simulink subsystem "Communication_Simulator"  (R2024a)
settings: Solver=VariableStepAuto  StartTime=0.0  StopTime=10.0  RelTol=1e-3
undefined symbols (not defined in the file): paramRFSatLink, QAM, rfSatSourceSamplesPerSymbol, rfSatSourceSampleTime
libraries: commrflib2 x24, dspsigops x12, commrfcorlib x8, commfilt2 x8, commdigbbndam3 x8, dspsolvers x8, simulink x8, commrandsrc3 x4, commsink2 x4, commdemoslib x4, impairlib x4, commsync2 x4
(part 1 of 3)
settings Model: Creator=dani  LastModifiedBy=dani

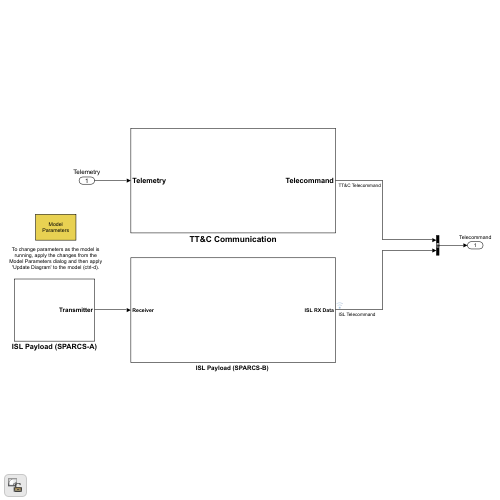
[thumbnail: Simulink's stored preview of the top-level diagram]
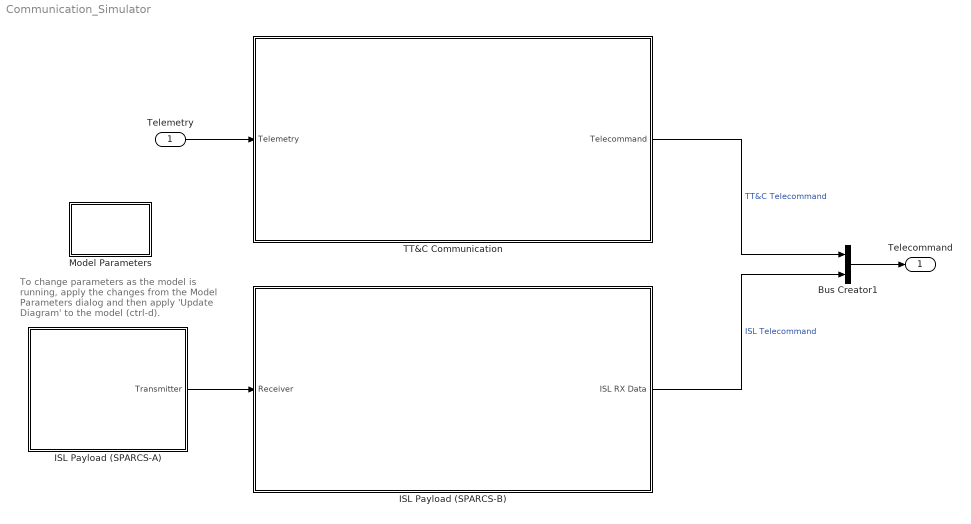
== system Communication_Simulator ==
  note: To change parameters as the model is running, apply the changes from the Model Parameters dialog and then apply 'Update Diagram' to the model (ctrl-d).
  Telemetry : Inport
  Bus Creator1 : BusCreator  Inputs=2
  ISL Payload (SPARCS-A) : Subsystem
  "ISL Payload (SPARCS-B) " : Subsystem
  Model Parameters : Subsystem  mask(Model Parameters){altitude=2500, frequency=435, antDiam=[.4 .4], selTemp=0 (no noise), selLvlBO=30 dB  (negligible nonlinearity), selDoppler=0 Hz, selNoPh=Negligible (-100 dBc/Hz @ 100 Hz), selImbal=None, selADC=No ADC, selPreDistortion=off, selDcOffset=off, selCorrIQ=off, selCorrDoppler=off}
      mask prompts: altitude "Satellite altitude (km):"; frequency "Frequency (MHz):"; antDiam "Transmit and receive antenna diameters (m):"; selTemp "Noise temperature (K):"; selLvlBO "HPA backoff level:"; selDoppler "Doppler error:"; selNoPh "Phase noise:"; selImbal "I/Q imbalance and DC offset:"; selADC "ADC:"; selPreDistortion "Digital predistortion"; selDcOffset "DC offset correction"; selCorrIQ "I/Q imbalance correction"; selCorrDoppler "Doppler correction"
      mask help:
      | Select the scenarios from the mask to change the link parameters. Each of the mask parameters sets the parameters in the corresponding RF impairment or corresponding correction block(s).
      |
      | To make changes as the model is running, apply the changes from this dialog and then apply Update Diagram to the model (crtl-d).
      mask init:
      | commrfsatlink_mask(selLvlBO,selTemp, ...
      |     selDoppler, selImbal, selNoPh, ...
      |     selDcOffset, selCorrDoppler, selCorrIQ, altitude, ...
      |     frequency, antDiam,8,6,selPreDistortion,selADC);
      mask Help: helpview(commdhelp);
      mask TypeOptions selTemp: 0 (no noise) | 20 (very low noise level) | 290 (typical noise level) | 500 (high noise level)
      mask TypeOptions selLvlBO: 30 dB  (negligible nonlinearity) | 7 dB  (moderate nonlinearity) | 1 dB  (severe nonlinearity)
      mask TypeOptions selDoppler: 0 Hz | 3 Hz
      mask TypeOptions selNoPh: Negligible (-100 dBc/Hz @ 100 Hz) | Low  (-55 dBc/Hz @ 100 Hz) | High  (-48 dBc/Hz @ 100 Hz)
      mask TypeOptions selImbal: None | Amplitude imbalance (3 dB) | Phase imbalance (20 deg) | In-phase DC offset (1e-8) | Quadrature DC offset (5e-8)
      mask TypeOptions selADC: No ADC | High resolution (16 bits) | Medium resolution (8 bits) | Low resolution (3 bits)
      mask Display: disp('Model\nParameters');
  TT&C Communication : Subsystem
  Telecommand : Outport
  wires:
  Bus Creator1/1 -> Telecommand/1
  TT&C Communication/1(Telecommand) -> Bus Creator1/1  "TT&C Telecommand"
  Telemetry/1 -> TT&C Communication/1(Telemetry)
  "ISL Payload (SPARCS-B) "/1(ISL RX Data) -> Bus Creator1/2  "ISL Telecommand"
  ISL Payload (SPARCS-A)/1(Transmitter) -> "ISL Payload (SPARCS-B) "/1(Receiver)

== system Communication_Simulator/ISL Payload (SPARCS-A) ==
  Bernoulli Binary Generator2 : commrandsrc3/Bernoulli Binary Generator  ProbabilityOfZero=0.5  SeedSource=Parameter  Seed=37  SampleTime=rfSatSourceSampleTime  SamplesPerFrame=rfSatSourceSamplesPerSymbol  OutputDataType=double  SimulateUsing=Interpreted execution
  Transmitter : Outport
  wires:
  Bernoulli Binary Generator2/1 -> Transmitter/1

== system Communication_Simulator/ISL Payload (SPARCS-B)  ==
  Receiver : Inport
  Display1 : Display
  ISL : Subsystem
  ISL RX Data : Outport
  wires:
  Receiver/1 -> ISL/1(isl_tx_data)
  ISL/1(isl_rx_data) -> ISL RX Data/1, Display1/1

== system Communication_Simulator/Model Parameters ==

== system Communication_Simulator/TT&C Communication ==
  Telemetry : Inport
  Bernoulli Binary Generator2 : commrandsrc3/Bernoulli Binary Generator  ProbabilityOfZero=0.5  SeedSource=Parameter  Seed=37  SampleTime=rfSatSourceSampleTime  SamplesPerFrame=rfSatSourceSamplesPerSymbol  OutputDataType=double  SimulateUsing=Interpreted execution
  Display : Display
  Ground Segment : Subsystem
  Terminator : Terminator
  Telecommand : Outport
  wires:
  Bernoulli Binary Generator2/1 -> Ground Segment/1(Telemetry)
  Telemetry/1 -> Terminator/1
  Ground Segment/1(Telecommand) -> Telecommand/1, Display/1

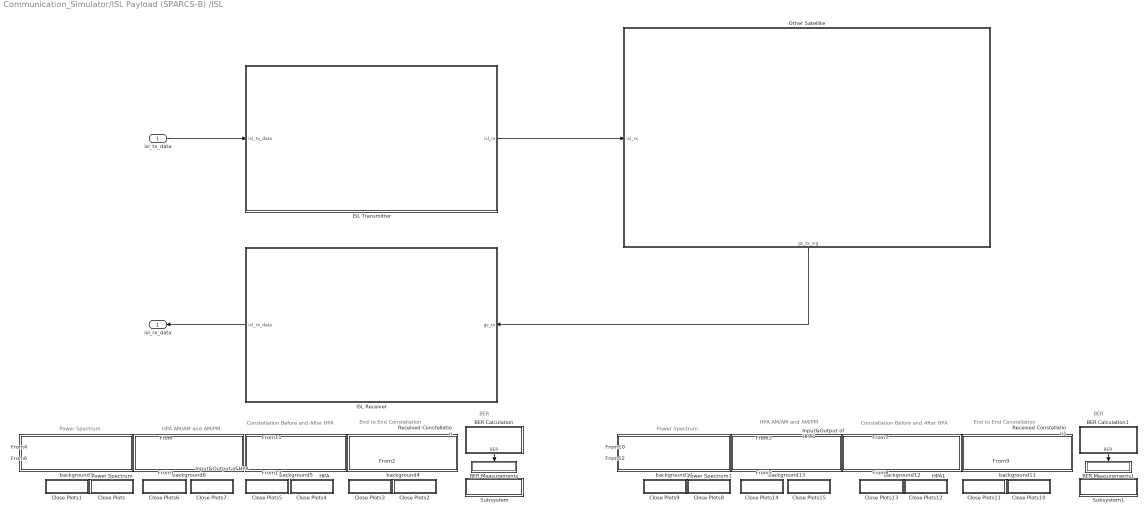
== system Communication_Simulator/ISL Payload (SPARCS-B) /ISL ==
  note: Constellation Before and
      | After HPA
  note: HPA AM/AM and AM/PM
  note: Power Spectrum
  note: BER
  note: End to End Constellation
  note: Power Spectrum
  note: BER
  note: Constellation Before and
      | After HPA
  note: End to End Constellation
  note: HPA AM/AM and AM/PM
  isl_tx_data : Inport
  BER Calculation : Subsystem
      mask Display: disp('Display Complete\nBit Error Rate\nInformation');
  BER Calculation1 : Subsystem
      mask Display: disp('Display Complete\nBit Error Rate\nInformation');
  BER Measurements : Display
      settings: Format=short_e
  BER Measurements1 : Display
      settings: Format=short_e
  Close Plots : Subsystem
      settings: OpenFcn=|
      | sdspfscope2([],[],[],'ScopeUpdate',[bdroot '/Power Spectrum/Tx and Rx Spectrum'],'CloseFig');
      | set_param([bdroot '/Power Spectrum/Tx and Rx Spectrum'],'OpenScopeAtSimStart','off');
      mask Display: disp('Close Scopes');
  Close Plots1 : Subsystem
      settings: OpenFcn=|
      | sdspfscope2([],[],[],'ScopeUpdate',[bdroot '/Power Spectrum/Tx and Rx Spectrum'],'OpenFig');
      | set_param([bdroot '/Power Spectrum/Tx and Rx Spectrum'],'OpenScopeAtSimStart','on');
      mask Display: disp('Open Scopes');
  Close Plots10 : Subsystem
      settings: OpenFcn=|
      | sdspfscope2([],[],[],'ScopeUpdate',[bdroot '/Received Constellation'],'CloseFig');
      |    set_param([bdroot '/Received Constellation'],'OpenScopeAtSimStart','off');
      mask Display: disp('Close Scopes');
  Close Plots11 : Subsystem
      settings: OpenFcn=|
      | sdspfscope2([],[],[],'ScopeUpdate',[bdroot '/Received Constellation'],'OpenFig');
      |     set_param([bdroot '/Received Constellation'],'OpenScopeAtSimStart','on');
      mask Display: disp('Open Scopes');
  Close Plots12 : Subsystem
      settings: OpenFcn=|
      | sdspfscope2([],[],[],'ScopeUpdate',[bdroot '/HPA/RRC signal before and after HPA'],'CloseFig');
      |   set_param([bdroot '/HPA/RRC signal before and after HPA'],'OpenScopeAtSimStart','off');
      mask Display: disp('Close Scopes');
  Close Plots13 : Subsystem
      settings: OpenFcn=|
      | sdspfscope2([],[],[],'ScopeUpdate',[bdroot '/HPA/RRC signal before and after HPA'],'OpenFig');
      | set_param([bdroot '/HPA/RRC signal before and after HPA'],'OpenScopeAtSimStart','on');
      mask Display: disp('Open Scopes');
  Close Plots14 : Subsystem
      settings: OpenFcn=|
      | sdspfscope2([],[],[],'ScopeUpdate',[bdroot '/Input&Output of HPA/HPA AM to AM'],'OpenFig');
      | set_param([bdroot '/Input&Output of HPA/HPA AM to AM'],'OpenScopeAtSimStart','on');
      | sdspfscope2([],[],[],'ScopeUpdate',[bdroot '/Input&Output of HPA/HPA AM to PM'],'OpenFig');
      | set_param([bdroot '/Input&Output of HPA/HPA AM to PM'],'OpenScopeAtSimStart','on');
      mask Display: disp('Open Scopes');
  Close Plots15 : Subsystem
      settings: OpenFcn=|
      | sdspfscope2([],[],[],'ScopeUpdate',[bdroot '/Input&Output of HPA/HPA AM to AM'],'CloseFig');
      | set_param([bdroot '/Input&Output of HPA/HPA AM to AM'],'OpenScopeAtSimStart','off');
      | sdspfscope2([],[],[],'ScopeUpdate',[bdroot '/Input&Output of HPA/HPA AM to PM'],'CloseFig');
      | set_param([bdroot '/Input&Output of HPA/HPA AM to PM'],'OpenScopeAtSimStart','off');
      mask Display: disp('Close Scopes');
  Close Plots2 : Subsystem
      settings: OpenFcn=|
      | sdspfscope2([],[],[],'ScopeUpdate',[bdroot '/Received Constellation'],'CloseFig');
      |    set_param([bdroot '/Received Constellation'],'OpenScopeAtSimStart','off');
      mask Display: disp('Close Scopes');
  Close Plots3 : Subsystem
      settings: OpenFcn=|
      | sdspfscope2([],[],[],'ScopeUpdate',[bdroot '/Received Constellation'],'OpenFig');
      |     set_param([bdroot '/Received Constellation'],'OpenScopeAtSimStart','on');
      mask Display: disp('Open Scopes');
  Close Plots4 : Subsystem
      settings: OpenFcn=|
      | sdspfscope2([],[],[],'ScopeUpdate',[bdroot '/HPA/RRC signal before and after HPA'],'CloseFig');
      |   set_param([bdroot '/HPA/RRC signal before and after HPA'],'OpenScopeAtSimStart','off');
      mask Display: disp('Close Scopes');
  Close Plots5 : Subsystem
      settings: OpenFcn=|
      | sdspfscope2([],[],[],'ScopeUpdate',[bdroot '/HPA/RRC signal before and after HPA'],'OpenFig');
      | set_param([bdroot '/HPA/RRC signal before and after HPA'],'OpenScopeAtSimStart','on');
      mask Display: disp('Open Scopes');
  Close Plots6 : Subsystem
      settings: OpenFcn=|
      | sdspfscope2([],[],[],'ScopeUpdate',[bdroot '/Input&Output of HPA/HPA AM to AM'],'OpenFig');
      | set_param([bdroot '/Input&Output of HPA/HPA AM to AM'],'OpenScopeAtSimStart','on');
      | sdspfscope2([],[],[],'ScopeUpdate',[bdroot '/Input&Output of HPA/HPA AM to PM'],'OpenFig');
      | set_param([bdroot '/Input&Output of HPA/HPA AM to PM'],'OpenScopeAtSimStart','on');
      mask Display: disp('Open Scopes');
  Close Plots7 : Subsystem
      settings: OpenFcn=|
      | sdspfscope2([],[],[],'ScopeUpdate',[bdroot '/Input&Output of HPA/HPA AM to AM'],'CloseFig');
      | set_param([bdroot '/Input&Output of HPA/HPA AM to AM'],'OpenScopeAtSimStart','off');
      | sdspfscope2([],[],[],'ScopeUpdate',[bdroot '/Input&Output of HPA/HPA AM to PM'],'CloseFig');
      | set_param([bdroot '/Input&Output of HPA/HPA AM to PM'],'OpenScopeAtSimStart','off');
      mask Display: disp('Close Scopes');
  Close Plots8 : Subsystem
      settings: OpenFcn=|
      | sdspfscope2([],[],[],'ScopeUpdate',[bdroot '/Power Spectrum/Tx and Rx Spectrum'],'CloseFig');
      | set_param([bdroot '/Power Spectrum/Tx and Rx Spectrum'],'OpenScopeAtSimStart','off');
      mask Display: disp('Close Scopes');
  Close Plots9 : Subsystem
      settings: OpenFcn=|
      | sdspfscope2([],[],[],'ScopeUpdate',[bdroot '/Power Spectrum/Tx and Rx Spectrum'],'OpenFig');
      | set_param([bdroot '/Power Spectrum/Tx and Rx Spectrum'],'OpenScopeAtSimStart','on');
      mask Display: disp('Open Scopes');
  HPA : Subsystem  TreatAsAtomicUnit=on
      mask Display: disp('HPA\nConstellation')
  HPA1 : Subsystem  TreatAsAtomicUnit=on
      mask Display: disp('HPA\nConstellation')
  ISL Receiver : Subsystem
  ISL Transmitter : Subsystem
  Input&Output of HPA : Subsystem
      mask Display: disp('Input/Output\nof HPA')
  Input&Output of HPA1 : Subsystem
      mask Display: disp('Input/Output\nof HPA')
  Other Satellite : Subsystem
      settings: PortSchema="{\"entries\":[{\"content\":{\"sides\":[{\"content\":{\"connectorIds\":[\"In1\"]},\"type\":\"ConnectorPlacement.EquallySpacedRectSide\",\"uuid\":\"5c052e88-5819-4bab-a9ca-1edf746c76a6\"},{\"content\":{\"side\":\"RIGHT\"},\"type\":\"ConnectorPlacement.EquallySpacedRectSide\",\"uuid\":\"3cddd3d4-de27-4776-a831-1e85d854be22\"},{\"content\":{\"side\":\"TOP\"},\"type\":\"ConnectorPlacement.EquallySpacedRectSide\",\"uuid\":\"b1cee8cc-56f8-4742-b35d-0b000ee97294\"},{\"content\":{\"connectorIds\":[\"Out1\"],\"side\":\"BOTTOM\"},\"type\":\"ConnectorPlacement.EquallySpacedRectSide\",\"uuid\":\"82960b08-fedb-40ff-a2ae-cc76727c9e64\"}]},\"type\":\"ConnectorPlacement.EquallySpacedConnector\",\"uuid\":\"cf72f4d7-97ef-46d7-aa70-0ebf7a9f667e\"}],\"packageUris\":[\"http://schema.mathworks.com/mf0/Connector/R2020b\"],\"version\":\"1.0\"}"
  Power Spectrum : Subsystem  TreatAsAtomicUnit=on
      mask Display: disp('Power\nSpectrum')
  Power Spectrum1 : Subsystem  TreatAsAtomicUnit=on
      mask Display: disp('Power\nSpectrum')
  Received Constellation : ConstellationDiagram  Tag=ScatterPlot  WindowPosition=[512.000000,233.000000,512.000000,399.000000,]  ScopeFrameLocation=window  SamplesPerSymbol=8  SymbolsToDisplaySource=Property  SymbolsToDisplay=1000  ReferenceConstellation="[-0.94868+0.94868i -0.94868+0.31623i -0.94868-0.94868i -0.94868-0.31623i -0.31623+0.94868i -0.31623+0.31623i -0.31623-0.94868i -0.31623-0.31623i  0.94868+0.94868i  0.94868+0.31623i  0.94868-0.94868i  0.94868-0.31623i  0.31623+0.94868i  0.31623+0.31623i  0.31623-0.94868i  0.31623-0.31623i]"  Title=Received Constellation  XLimits=[-1.5 1.5]  YLimits=[-1.5 1.5]  ColorFading=on  DefaultConfigurationName=comm.scopes.ConstellationDiagramBlockCfg
  Received Constellation1 : ConstellationDiagram  Tag=ScatterPlot  WindowPosition=[886 364 270 242]  SamplesPerSymbol=8  SymbolsToDisplaySource=Property  SymbolsToDisplay=1000  ReferenceConstellation="[-0.94868+0.94868i -0.94868+0.31623i -0.94868-0.94868i -0.94868-0.31623i -0.31623+0.94868i -0.31623+0.31623i -0.31623-0.94868i -0.31623-0.31623i  0.94868+0.94868i  0.94868+0.31623i  0.94868-0.94868i  0.94868-0.31623i  0.31623+0.94868i  0.31623+0.31623i  0.31623-0.94868i  0.31623-0.31623i]"  Title=Received Constellation  XLimits=[-1.5 1.5]  YLimits=[-1.5 1.5]  ColorFading=on  DefaultConfigurationName=comm.scopes.ConstellationDiagramBlockCfg
      settings: OpenAtSimulationStart=off
  Subsystem : Subsystem
      settings: OpenFcn=|
      | % Set value to reset BER
      | warning('off', 'Simulink:Engine:NonTunableVarChanged');
      | paramRFSatLink.resetBER = 1;
      | set_param(bdroot, 'SimulationCommand', 'update');
      | pause(0.1)
      | 
      | % Set value so that BER is not continually reset
      | paramRFSatLink.resetBER = 0;
      | set_param(bdroot, 'SimulationCommand', 'update');
      | warning('on', 'Simulink:Engine:NonTunableVarChanged');
      mask Display: disp('Double-click to\nreset BER')
  Subsystem1 : Subsystem
      settings: OpenFcn=|
      | % Set value to reset BER
      | warning('off', 'Simulink:Engine:NonTunableVarChanged');
      | paramRFSatLink.resetBER = 1;
      | set_param(bdroot, 'SimulationCommand', 'update');
      | pause(0.1)
      | 
      | % Set value so that BER is not continually reset
      | paramRFSatLink.resetBER = 0;
      | set_param(bdroot, 'SimulationCommand', 'update');
      | warning('on', 'Simulink:Engine:NonTunableVarChanged');
      mask Display: disp('Double-click to\nreset BER')
  background11 : Subsystem
      mask Display: disp('')
  background12 : Subsystem
      mask Display: disp('')
  background13 : Subsystem
      mask Display: disp('')
  background14 : Subsystem
      mask Display: disp('')
  background4 : Subsystem
      mask Display: disp('')
  background5 : Subsystem
      mask Display: disp('')
  background6 : Subsystem
      mask Display: disp('')
  background7 : Subsystem
      mask Display: disp('')
  isl_rx_data : Outport
  wires:
  [Rx_isl_RRC] -> Power Spectrum/2(In2)
  [HPA_Out_isl] -> Input&Output of HPA/2(In2)
  [Rx__isl_Const] -> Received Constellation/1
  [HPA_In_isl] -> Input&Output of HPA/1(In1)
  [Tx_isl_RRC] -> Power Spectrum/1(In1)
  BER Calculation/1(BER) -> BER Measurements/1
  [Tx_isl_Ampl_Return] -> HPA1/1(HPA Input)
  [Tx_isl_Ampl] -> HPA/2(HPA Output)
  [Rx_isl_RRC_Return] -> Power Spectrum1/2(In2)
  BER Calculation1/1(BER) -> BER Measurements1/1
  [HPA_In_isl_Return] -> Input&Output of HPA1/1(In1)
  [Rx_isl_RRC_Return] -> HPA1/2(HPA Output)
  [HPA_Out_isl_Return] -> Input&Output of HPA1/2(In2)
  [Tx_isl_RRC_Return] -> Power Spectrum1/1(In1)
  [Rx_isl_RRC] -> HPA/1(HPA Input)
  [Rx__isl_Const_Return] -> Received Constellation1/1
  ISL Receiver/1(isl_rx_data) -> isl_rx_data/1
  ISL Transmitter/1(isl_rx) -> Other Satellite/1(isl_rx)
  Other Satellite/1(gs_tx_sig) -> ISL Receiver/1(gs_tx)
  isl_tx_data/1 -> ISL Transmitter/1(isl_tx_data)

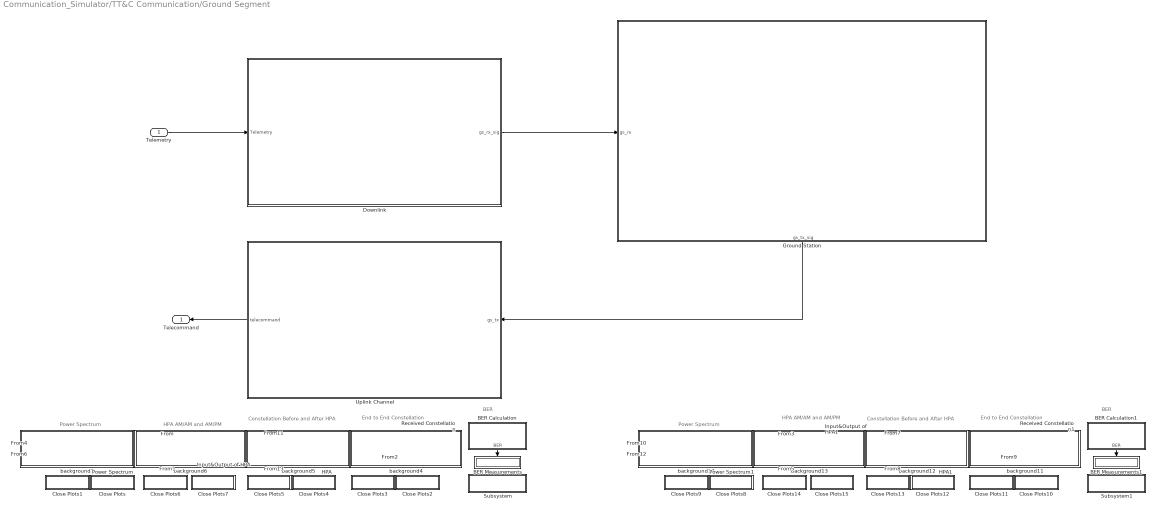
== system Communication_Simulator/TT&C Communication/Ground Segment ==
  note: Constellation Before and
      | After HPA
  note: HPA AM/AM and AM/PM
  note: Power Spectrum
  note: BER
  note: End to End Constellation
  note: Power Spectrum
  note: BER
  note: Constellation Before and
      | After HPA
  note: End to End Constellation
  note: HPA AM/AM and AM/PM
  Telemetry : Inport
  BER Calculation : Subsystem
      mask Display: disp('Display Complete\nBit Error Rate\nInformation');
  BER Calculation1 : Subsystem
      mask Display: disp('Display Complete\nBit Error Rate\nInformation');
  BER Measurements : Display
      settings: Format=short_e
  BER Measurements1 : Display
      settings: Format=short_e
  Close Plots : Subsystem
      settings: OpenFcn=|
      | sdspfscope2([],[],[],'ScopeUpdate',[bdroot '/Power Spectrum/Tx and Rx Spectrum'],'CloseFig');
      | set_param([bdroot '/Power Spectrum/Tx and Rx Spectrum'],'OpenScopeAtSimStart','off');
      mask Display: disp('Close Scopes');
  Close Plots1 : Subsystem
      settings: OpenFcn=|
      | sdspfscope2([],[],[],'ScopeUpdate',[bdroot '/Power Spectrum/Tx and Rx Spectrum'],'OpenFig');
      | set_param([bdroot '/Power Spectrum/Tx and Rx Spectrum'],'OpenScopeAtSimStart','on');
      mask Display: disp('Open Scopes');
  Close Plots10 : Subsystem
      settings: OpenFcn=|
      | sdspfscope2([],[],[],'ScopeUpdate',[bdroot '/Received Constellation'],'CloseFig');
      |    set_param([bdroot '/Received Constellation'],'OpenScopeAtSimStart','off');
      mask Display: disp('Close Scopes');
  Close Plots11 : Subsystem
      settings: OpenFcn=|
      | sdspfscope2([],[],[],'ScopeUpdate',[bdroot '/Received Constellation'],'OpenFig');
      |     set_param([bdroot '/Received Constellation'],'OpenScopeAtSimStart','on');
      mask Display: disp('Open Scopes');
  Close Plots12 : Subsystem
      settings: OpenFcn=|
      | sdspfscope2([],[],[],'ScopeUpdate',[bdroot '/HPA/RRC signal before and after HPA'],'CloseFig');
      |   set_param([bdroot '/HPA/RRC signal before and after HPA'],'OpenScopeAtSimStart','off');
      mask Display: disp('Close Scopes');
  Close Plots13 : Subsystem
      settings: OpenFcn=|
      | sdspfscope2([],[],[],'ScopeUpdate',[bdroot '/HPA/RRC signal before and after HPA'],'OpenFig');
      | set_param([bdroot '/HPA/RRC signal before and after HPA'],'OpenScopeAtSimStart','on');
      mask Display: disp('Open Scopes');
  Close Plots14 : Subsystem
      settings: OpenFcn=|
      | sdspfscope2([],[],[],'ScopeUpdate',[bdroot '/Input&Output of HPA/HPA AM to AM'],'OpenFig');
      | set_param([bdroot '/Input&Output of HPA/HPA AM to AM'],'OpenScopeAtSimStart','on');
      | sdspfscope2([],[],[],'ScopeUpdate',[bdroot '/Input&Output of HPA/HPA AM to PM'],'OpenFig');
      | set_param([bdroot '/Input&Output of HPA/HPA AM to PM'],'OpenScopeAtSimStart','on');
      mask Display: disp('Open Scopes');
  Close Plots15 : Subsystem
      settings: OpenFcn=|
      | sdspfscope2([],[],[],'ScopeUpdate',[bdroot '/Input&Output of HPA/HPA AM to AM'],'CloseFig');
      | set_param([bdroot '/Input&Output of HPA/HPA AM to AM'],'OpenScopeAtSimStart','off');
      | sdspfscope2([],[],[],'ScopeUpdate',[bdroot '/Input&Output of HPA/HPA AM to PM'],'CloseFig');
      | set_param([bdroot '/Input&Output of HPA/HPA AM to PM'],'OpenScopeAtSimStart','off');
      mask Display: disp('Close Scopes');
  Close Plots2 : Subsystem
      settings: OpenFcn=|
      | sdspfscope2([],[],[],'ScopeUpdate',[bdroot '/Received Constellation'],'CloseFig');
      |    set_param([bdroot '/Received Constellation'],'OpenScopeAtSimStart','off');
      mask Display: disp('Close Scopes');
  Close Plots3 : Subsystem
      settings: OpenFcn=|
      | sdspfscope2([],[],[],'ScopeUpdate',[bdroot '/Received Constellation'],'OpenFig');
      |     set_param([bdroot '/Received Constellation'],'OpenScopeAtSimStart','on');
      mask Display: disp('Open Scopes');
  Close Plots4 : Subsystem
      settings: OpenFcn=|
      | sdspfscope2([],[],[],'ScopeUpdate',[bdroot '/HPA/RRC signal before and after HPA'],'CloseFig');
      |   set_param([bdroot '/HPA/RRC signal before and after HPA'],'OpenScopeAtSimStart','off');
      mask Display: disp('Close Scopes');
  Close Plots5 : Subsystem
      settings: OpenFcn=|
      | sdspfscope2([],[],[],'ScopeUpdate',[bdroot '/HPA/RRC signal before and after HPA'],'OpenFig');
      | set_param([bdroot '/HPA/RRC signal before and after HPA'],'OpenScopeAtSimStart','on');
      mask Display: disp('Open Scopes');
  Close Plots6 : Subsystem
      settings: OpenFcn=|
      | sdspfscope2([],[],[],'ScopeUpdate',[bdroot '/Input&Output of HPA/HPA AM to AM'],'OpenFig');
      | set_param([bdroot '/Input&Output of HPA/HPA AM to AM'],'OpenScopeAtSimStart','on');
      | sdspfscope2([],[],[],'ScopeUpdate',[bdroot '/Input&Output of HPA/HPA AM to PM'],'OpenFig');
      | set_param([bdroot '/Input&Output of HPA/HPA AM to PM'],'OpenScopeAtSimStart','on');
      mask Display: disp('Open Scopes');
  Close Plots7 : Subsystem
      settings: OpenFcn=|
      | sdspfscope2([],[],[],'ScopeUpdate',[bdroot '/Input&Output of HPA/HPA AM to AM'],'CloseFig');
      | set_param([bdroot '/Input&Output of HPA/HPA AM to AM'],'OpenScopeAtSimStart','off');
      | sdspfscope2([],[],[],'ScopeUpdate',[bdroot '/Input&Output of HPA/HPA AM to PM'],'CloseFig');
      | set_param([bdroot '/Input&Output of HPA/HPA AM to PM'],'OpenScopeAtSimStart','off');
      mask Display: disp('Close Scopes');
  Close Plots8 : Subsystem
      settings: OpenFcn=|
      | sdspfscope2([],[],[],'ScopeUpdate',[bdroot '/Power Spectrum/Tx and Rx Spectrum'],'CloseFig');
      | set_param([bdroot '/Power Spectrum/Tx and Rx Spectrum'],'OpenScopeAtSimStart','off');
      mask Display: disp('Close Scopes');
  Close Plots9 : Subsystem
      settings: OpenFcn=|
      | sdspfscope2([],[],[],'ScopeUpdate',[bdroot '/Power Spectrum/Tx and Rx Spectrum'],'OpenFig');
      | set_param([bdroot '/Power Spectrum/Tx and Rx Spectrum'],'OpenScopeAtSimStart','on');
      mask Display: disp('Open Scopes');
  Downlink : Subsystem
  Ground Station : Subsystem
      settings: PortSchema="{\"entries\":[{\"content\":{\"sides\":[{\"content\":{\"connectorIds\":[\"In1\"]},\"type\":\"ConnectorPlacement.EquallySpacedRectSide\",\"uuid\":\"5c052e88-5819-4bab-a9ca-1edf746c76a6\"},{\"content\":{\"side\":\"RIGHT\"},\"type\":\"ConnectorPlacement.EquallySpacedRectSide\",\"uuid\":\"3cddd3d4-de27-4776-a831-1e85d854be22\"},{\"content\":{\"side\":\"TOP\"},\"type\":\"ConnectorPlacement.EquallySpacedRectSide\",\"uuid\":\"b1cee8cc-56f8-4742-b35d-0b000ee97294\"},{\"content\":{\"connectorIds\":[\"Out1\"],\"side\":\"BOTTOM\"},\"type\":\"ConnectorPlacement.EquallySpacedRectSide\",\"uuid\":\"82960b08-fedb-40ff-a2ae-cc76727c9e64\"}]},\"type\":\"ConnectorPlacement.EquallySpacedConnector\",\"uuid\":\"cf72f4d7-97ef-46d7-aa70-0ebf7a9f667e\"}],\"packageUris\":[\"http://schema.mathworks.com/mf0/Connector/R2020b\"],\"version\":\"1.0\"}"
  HPA : Subsystem  TreatAsAtomicUnit=on
      mask Display: disp('HPA\nConstellation')
  HPA1 : Subsystem  TreatAsAtomicUnit=on
      mask Display: disp('HPA\nConstellation')
  Input&Output of HPA : Subsystem
      mask Display: disp('Input/Output\nof HPA')
  Input&Output of HPA1 : Subsystem
      mask Display: disp('Input/Output\nof HPA')
  Power Spectrum : Subsystem  TreatAsAtomicUnit=on
      mask Display: disp('Power\nSpectrum')
  Power Spectrum1 : Subsystem  TreatAsAtomicUnit=on
      mask Display: disp('Power\nSpectrum')
  Received Constellation : ConstellationDiagram  Tag=ScatterPlot  WindowPosition=[1024.000000,41.000000,516.000000,364.000000,]  ScopeFrameLocation=window  SamplesPerSymbol=8  SymbolsToDisplaySource=Property  SymbolsToDisplay=1000  ReferenceConstellation="[-0.94868+0.94868i -0.94868+0.31623i -0.94868-0.94868i -0.94868-0.31623i -0.31623+0.94868i -0.31623+0.31623i -0.31623-0.94868i -0.31623-0.31623i  0.94868+0.94868i  0.94868+0.31623i  0.94868-0.94868i  0.94868-0.31623i  0.31623+0.94868i  0.31623+0.31623i  0.31623-0.94868i  0.31623-0.31623i]"  Title=Received Constellation  XLimits=[-1.5 1.5]  YLimits=[-1.5 1.5]  ColorFading=on  DefaultConfigurationName=comm.scopes.ConstellationDiagramBlockCfg
  Received Constellation1 : ConstellationDiagram  Tag=ScatterPlot  WindowPosition=[886 364 270 242]  SamplesPerSymbol=8  SymbolsToDisplaySource=Property  SymbolsToDisplay=1000  ReferenceConstellation="[-0.94868+0.94868i -0.94868+0.31623i -0.94868-0.94868i -0.94868-0.31623i -0.31623+0.94868i -0.31623+0.31623i -0.31623-0.94868i -0.31623-0.31623i  0.94868+0.94868i  0.94868+0.31623i  0.94868-0.94868i  0.94868-0.31623i  0.31623+0.94868i  0.31623+0.31623i  0.31623-0.94868i  0.31623-0.31623i]"  Title=Received Constellation  XLimits=[-1.5 1.5]  YLimits=[-1.5 1.5]  ColorFading=on  DefaultConfigurationName=comm.scopes.ConstellationDiagramBlockCfg
      settings: OpenAtSimulationStart=off
  Subsystem : Subsystem
      settings: OpenFcn=|
      | % Set value to reset BER
      | warning('off', 'Simulink:Engine:NonTunableVarChanged');
      | paramRFSatLink.resetBER = 1;
      | set_param(bdroot, 'SimulationCommand', 'update');
      | pause(0.1)
      | 
      | % Set value so that BER is not continually reset
      | paramRFSatLink.resetBER = 0;
      | set_param(bdroot, 'SimulationCommand', 'update');
      | warning('on', 'Simulink:Engine:NonTunableVarChanged');
      mask Display: disp('Double-click to\nreset BER')
  Subsystem1 : Subsystem
      settings: OpenFcn=|
      | % Set value to reset BER
      | warning('off', 'Simulink:Engine:NonTunableVarChanged');
      | paramRFSatLink.resetBER = 1;
      | set_param(bdroot, 'SimulationCommand', 'update');
      | pause(0.1)
      | 
      | % Set value so that BER is not continually reset
      | paramRFSatLink.resetBER = 0;
      | set_param(bdroot, 'SimulationCommand', 'update');
      | warning('on', 'Simulink:Engine:NonTunableVarChanged');
      mask Display: disp('Double-click to\nreset BER')
  Uplink Channel : Subsystem
  background11 : Subsystem
      mask Display: disp('')
  background12 : Subsystem
      mask Display: disp('')
  background13 : Subsystem
      mask Display: disp('')
  background14 : Subsystem
      mask Display: disp('')
  background4 : Subsystem
      mask Display: disp('')
  background5 : Subsystem
      mask Display: disp('')
  background6 : Subsystem
      mask Display: disp('')
  background7 : Subsystem
      mask Display: disp('')
  Telecommand : Outport
  wires:
  [Rx_downlink_RRC] -> Power Spectrum/2(In2)
  [HPA_Out_downlink] -> Input&Output of HPA/2(In2)
  [Rx__downlink_Const] -> Received Constellation/1
  [HPA_In_downlink] -> Input&Output of HPA/1(In1)
  [Tx_downlink_RRC] -> Power Spectrum/1(In1)
  BER Calculation/1(BER) -> BER Measurements/1
  [Tx_uplink_Ampl] -> HPA1/1(HPA Input)
  [Tx_downlink_Ampl] -> HPA/2(HPA Output)
  [Rx_uplink_RRC] -> Power Spectrum1/2(In2)
  BER Calculation1/1(BER) -> BER Measurements1/1
  [HPA_In_uplink] -> Input&Output of HPA1/1(In1)
  [Rx_uplink_RRC] -> HPA1/2(HPA Output)
  [HPA_Out_uplink] -> Input&Output of HPA1/2(In2)
  [Tx_uplink_RRC] -> Power Spectrum1/1(In1)
  [Rx_downlink_RRC] -> HPA/1(HPA Input)
  [Rx__uplink_Const] -> Received Constellation1/1
  Uplink Channel/1(telecommand) -> Telecommand/1
  Downlink/1(gs_rx_sig) -> Ground Station/1(gs_rx)
  Ground Station/1(gs_tx_sig) -> Uplink Channel/1(gs_tx)
  Telemetry/1 -> Downlink/1(Telemetry)

== system Communication_Simulator/ISL Payload (SPARCS-B) /ISL/BER Calculation ==
  note: BER Results (with reset)
  note: Bits
  note: Errors
  note: BER
  BER Measurements : Display
  Constant : Constant  Value=paramRFSatLink.resetBER  SampleTime=rfSatSourceSampleTime * rfSatSourceSamplesPerSymbol
  Error Rate Calculation : commsink2/Error Rate Calculation  N=24  st_delay=0  cp_mode=Entire frame  subframe=[]  PMode=Port  WsName=ErrorVec  RsMode2=on  stop=off  numErr=200  maxBits=1e6
  Selector : Selector  InputPortWidth=3  IndexOptions=Index vector (dialog)  Indices=[1]  OutputSizes=1
  BER : Outport  VectorParamsAs1DForOutWhenUnconnected=off
  wires:
  [RF_isl_Tx] -> Error Rate Calculation/1
  Selector/1 -> BER/1
  Constant/1 -> Error Rate Calculation/3
  Error Rate Calculation/1 -> BER Measurements/1, Selector/1
  [RF_isl_Rx] -> Error Rate Calculation/2

== system Communication_Simulator/ISL Payload (SPARCS-B) /ISL/BER Calculation1 ==
  note: BER Results (with reset)
  note: Bits
  note: Errors
  note: BER
  BER Measurements : Display
  Constant : Constant  Value=paramRFSatLink.resetBER  SampleTime=rfSatSourceSampleTime * rfSatSourceSamplesPerSymbol
  Error Rate Calculation : commsink2/Error Rate Calculation  N=24  st_delay=0  cp_mode=Entire frame  subframe=[]  PMode=Port  WsName=ErrorVec  RsMode2=on  stop=off  numErr=200  maxBits=1e6
  Selector : Selector  InputPortWidth=3  IndexOptions=Index vector (dialog)  Indices=[1]  OutputSizes=1
  BER : Outport  VectorParamsAs1DForOutWhenUnconnected=off
  wires:
  [RF_isl_Tx_Return] -> Error Rate Calculation/1
  Selector/1 -> BER/1
  Constant/1 -> Error Rate Calculation/3
  Error Rate Calculation/1 -> BER Measurements/1, Selector/1
  [RF_isl_Rx_Return] -> Error Rate Calculation/2

== system Communication_Simulator/ISL Payload (SPARCS-B) /ISL/Close Plots ==

== system Communication_Simulator/ISL Payload (SPARCS-B) /ISL/Close Plots1 ==

== system Communication_Simulator/ISL Payload (SPARCS-B) /ISL/Close Plots10 ==

== system Communication_Simulator/ISL Payload (SPARCS-B) /ISL/Close Plots11 ==

== system Communication_Simulator/ISL Payload (SPARCS-B) /ISL/Close Plots12 ==

== system Communication_Simulator/ISL Payload (SPARCS-B) /ISL/Close Plots13 ==

== system Communication_Simulator/ISL Payload (SPARCS-B) /ISL/Close Plots14 ==

== system Communication_Simulator/ISL Payload (SPARCS-B) /ISL/Close Plots15 ==

== system Communication_Simulator/ISL Payload (SPARCS-B) /ISL/Close Plots2 ==

== system Communication_Simulator/ISL Payload (SPARCS-B) /ISL/Close Plots3 ==

== system Communication_Simulator/ISL Payload (SPARCS-B) /ISL/Close Plots4 ==

== system Communication_Simulator/ISL Payload (SPARCS-B) /ISL/Close Plots5 ==

== system Communication_Simulator/ISL Payload (SPARCS-B) /ISL/Close Plots6 ==

== system Communication_Simulator/ISL Payload (SPARCS-B) /ISL/Close Plots7 ==

== system Communication_Simulator/ISL Payload (SPARCS-B) /ISL/Close Plots8 ==

== system Communication_Simulator/ISL Payload (SPARCS-B) /ISL/Close Plots9 ==

== system Communication_Simulator/ISL Payload (SPARCS-B) /ISL/HPA ==
  HPA Input : Inport
  HPA Output : Inport  Port=2
  Matrix Concatenate : Concatenate  Mode=Multidimensional array  ConcatenateDimension=2
  RRC signal before and after HPA : ConstellationDiagram  WindowPosition=[508.333333333333 347.666666666667 282 242.666666666667]  SamplesPerSymbol=8  SymbolsToDisplaySource=Property  SymbolsToDisplay=1000  ReferenceConstellation=16-QAM  Title=RRC Signal Before and After HPA  XLimits=[-3.9233 3.9259]  YLimits=[-3.9233 3.9259]  ShowLegend=on  ShowReferenceConstellation=off  ColorFading=on  DefaultConfigurationName=comm.scopes.ConstellationDiagramBlockCfg
      settings: OpenAtSimulationStart=off
  wires:
  Matrix Concatenate/1 -> RRC signal before and after HPA/1
  HPA Output/1 -> Matrix Concatenate/2
  HPA Input/1 -> Matrix Concatenate/1

== system Communication_Simulator/ISL Payload (SPARCS-B) /ISL/HPA1 ==
  HPA Input : Inport
  HPA Output : Inport  Port=2
  Matrix Concatenate : Concatenate  Mode=Multidimensional array  ConcatenateDimension=2
  RRC signal before and after HPA : ConstellationDiagram  WindowPosition=[508.333333333333 347.666666666667 282 242.666666666667]  SamplesPerSymbol=8  SymbolsToDisplaySource=Property  SymbolsToDisplay=1000  ReferenceConstellation=16-QAM  Title=RRC Signal Before and After HPA  XLimits=[-3.9233 3.9259]  YLimits=[-3.9233 3.9259]  ShowLegend=on  ShowReferenceConstellation=off  ColorFading=on  DefaultConfigurationName=comm.scopes.ConstellationDiagramBlockCfg
      settings: OpenAtSimulationStart=off
  wires:
  Matrix Concatenate/1 -> RRC signal before and after HPA/1
  HPA Output/1 -> Matrix Concatenate/2
  HPA Input/1 -> Matrix Concatenate/1

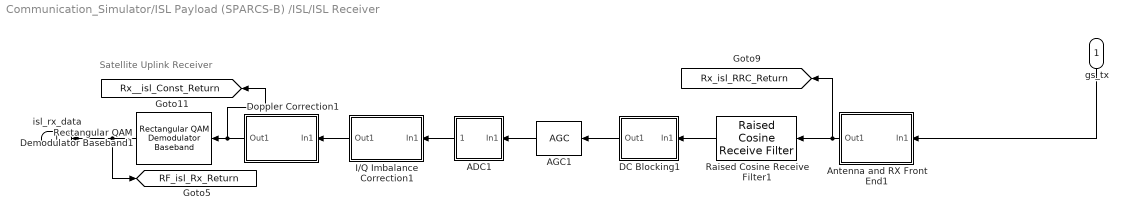
== system Communication_Simulator/ISL Payload (SPARCS-B) /ISL/ISL Receiver ==
  note: Satellite Uplink Receiver
  gs_tx : Inport
  ADC1 : Subsystem
      mask Display: disp('Bipolar\nADC')
  AGC1 : commrfcorlib/AGC  LegacyMode=off  DetectorMethod=Rectifier  LoopMethod=Linear  UpdatePeriod=100  StepSize=0.1  AdaptationStepSize=0.01  DesiredOutputPower=1  AveragingLength=256  MaximumGain=30  MaxPowerGain=400  GainOutputPort=off  InputPowerOutputPort=off  SimulateUsing=Code generation
  Antenna and RX Front End1 : Subsystem
      mask Display: disp('Antenna\nand\nRX Front End')
  DC Blocking1 : Subsystem
      mask Display: disp('DC\nBlocking')
  Doppler Correction1 : Subsystem
      mask Display: disp('Doppler\nCorrection')
  I/Q Imbalance Correction1 : Subsystem
      mask Display: disp('I/Q Imbalance\nCorrection')
  Raised Cosine Receive Filter1 : commfilt2/Raised Cosine Receive Filter  filtType=Square root  R=0.3  filtSpan=paramRFSatLink.FilterSpan  N=paramRFSatLink.SamplesPerSymbol  downFactor=paramRFSatLink.SamplesPerSymbol  downOffset=0  filterGain=1/sqrt(paramRFSatLink.SamplesPerSymbol)  InputProcessing=Columns as channels (frame based)  RateOptions=Enforce single-rate processing  framing=Mute  checkCoeff=off  variableName=rcRxFilt1  currentFiltSpan=2*((2*(3))/2)  D=(2*(3))/2  inputOffset=0  sampMode=Mute  saveAsFlag=0  rateMode=Downsampling  checkGain=Normalized  launchFVT=off  roundingMode=Floor  overflowMode=off  coeffDataTypeStr=Inherit: Same word length as input  coeffMin=[]  coeffMax=[]  coeffLastDataTypeStr=Inherit: Same word length as input  accumDataTypeStr=Inherit: Same as product output  accumLastDataTypeStr=Inherit: Same as product output  outputDataTypeStr=Inherit: Same as accumulator  outputMin=[]  outputMax=[]  outputLastDataTypeStr=Inherit: Same as accumulator
  Rectangular QAM Demodulator Baseband1 : commdigbbndam3/Rectangular QAM Demodulator Baseband  M=16  OutType=Bit  DecType=Hard decision  VarSource=Dialog  Variance=1  Dec=Gray  Mapping=[0:15]  PowType=Average Power  MinDist=2  AvgPow=1  PeakPow=1  Ph=0  outDtype1=double  outDtype2=double  derotateFactorWordLen=16  derotateFactorDataTypeStr=Inherit: Same word length as input  derotateFactorLastDataTypeStr=Inherit: Same word length as input  denormFactorWordLen=16  denormFactorDataTypeStr=Inherit: Same word length as input  denormFactorLastDataTypeStr=Inherit: Same word length as input  prodOutWordLen=32  prodOutOverflowMode=Wrap  prodOutRoundingMode=Floor  prodOutOvFlMode=off  prodOutOvFlModeLastStrValue=off  sumWordLen=32
  isl_rx_data : Outport
  tag scope: RF_isl_Rx_Return=global, Rx__isl_Const_Return=global, Rx_isl_RRC_Return=global
  wires:
  gs_tx/1 -> Antenna and RX Front End1/1(In1)
  I/Q Imbalance Correction1/1(Out1) -> Doppler Correction1/1(In1)
  Rectangular QAM Demodulator Baseband1/1 -> [RF_isl_Rx_Return], isl_rx_data/1
  AGC1/1 -> ADC1/1(In1)
  Raised Cosine Receive Filter1/1 -> DC Blocking1/1(In1)
  ADC1/1(Out2) -> I/Q Imbalance Correction1/1(In1)
  Antenna and RX Front End1/1(Out1) -> [Rx_isl_RRC_Return], Raised Cosine Receive Filter1/1
  Doppler Correction1/1(Out1) -> Rectangular QAM Demodulator Baseband1/1, [Rx__isl_Const_Return]
  DC Blocking1/1(Out1) -> AGC1/1

== system Communication_Simulator/ISL Payload (SPARCS-B) /ISL/ISL Transmitter ==
  note: ISL Transmitter
  note: Transmitter
  isl_tx_data : Inport
  Doppler Error : commrflib2/Phase// Frequency Offset  phaseOffset=0  freqPort=off  freqOffset=paramRFSatLink.DoppOffset
  Downlink Path : commrflib2/Free Space Path Loss  mode=Distance and Frequency  dB=180  d=paramRFSatLink.Altitude  fc=paramRFSatLink.Frequency
  Nonlinearity : Subsystem
      mask Display: disp('HPA\n Nonlinearity\n with Optional\n Digital\nPredistortion')
  Raised Cosine Transmit Filter : commfilt2/Raised Cosine Transmit Filter  filtType=Square root  R=0.3  filtSpan=paramRFSatLink.FilterSpan  N=paramRFSatLink.SamplesPerSymbol  filterGain=sqrt(paramRFSatLink.SamplesPerSymbol)  InputProcessing=Columns as channels (frame based)  RateOptions=Enforce single-rate processing  framing=Mute  checkCoeff=off  variableName=rcTxFilt  checkGain=Normalized  sampMode=Mute  saveAsFlag=0  currentFiltSpan=2*((2*(3))/2)  D=(2*(3))/2  launchFVT=off  roundingMode=Floor  overflowMode=off  coeffDataTypeStr=Inherit: Same word length as input  coeffMin=[]  coeffMax=[]  coeffLastDataTypeStr=Inherit: Same word length as input  outputDataTypeStr=Inherit: Same as accumulator  outputMin=[]  outputMax=[]  outputLastDataTypeStr=Inherit: Same as accumulator
  Rectangular QAM Modulator Baseband : commdigbbndam3/Rectangular QAM Modulator Baseband  M=16  InType=Bit  Enc=Gray  Mapping=[0:15]  PowType=Average Power  MinDist=2  AvgPow=2  PeakPow=1  Ph=0  outDtype=double  outWordLen=16  outUDDataType=sfix(16)  outFracLenMode=Best precision  outFracLen=15  outDataTypeStr=double  outLastDataTypeStr=double
  Tx Dish Antenna Gain : Gain  Gain=paramRFSatLink.TXAntGain_ISL  SaturateOnIntegerOverflow=on  OutDataTypeStr=Inherit: Same as input  ParamDataTypeStr=Inherit: Same as input
  isl_rx : Outport
  tag scope: RF_isl_Tx=global, Tx_isl_Ampl=global, Tx_isl_RRC=global
  wires:
  Tx Dish Antenna Gain/1 -> Downlink Path/1
  Downlink Path/1 -> Doppler Error/1
  Doppler Error/1 -> isl_rx/1
  isl_tx_data/1 -> [RF_isl_Tx], Rectangular QAM Modulator Baseband/1
  Nonlinearity/1(Out2) -> Tx Dish Antenna Gain/1, [Tx_isl_Ampl]
  Rectangular QAM Modulator Baseband/1 -> Raised Cosine Transmit Filter/1
  Raised Cosine Transmit Filter/1 -> Nonlinearity/1(In), [Tx_isl_RRC]

== system Communication_Simulator/ISL Payload (SPARCS-B) /ISL/Input&Output of HPA ==
  In1 : Inport
  In2 : Inport  Port=2
  Add : Sum  Inputs=-+
  Complex to Magnitude-Angle : ComplexToMagnitudeAngle
  Complex to Magnitude-Angle1 : ComplexToMagnitudeAngle
  HPA AM to AM : ConstellationDiagram  Tag=ScatterPlot  WindowPosition=[1104 604 253 220]  SymbolsToDisplaySource=Property  SymbolsToDisplay=1000  Title=HPA AM to AM  XLimits=[-1.4713 6.1709]  YLimits=[-1.4713 6.1709]  XLabel=Input Amplitude  YLabel=Output Amplitude  ShowReferenceConstellation=off  ColorFading=on  DefaultConfigurationName=comm.scopes.ConstellationDiagramBlockCfg
      settings: OpenAtSimulationStart=off
  HPA AM to PM : ConstellationDiagram  Tag=ScatterPlot  WindowPosition=[842 605 253 220]  SymbolsToDisplaySource=Property  SymbolsToDisplay=1000  Title=HPA AM to PM  XLimits=[-1.0435 2.3201]  YLimits=[-1.0435 2.3201]  XLabel=Input Amplitude  YLabel=Phase Difference (rad)  ShowReferenceConstellation=off  ColorFading=on  DefaultConfigurationName=comm.scopes.ConstellationDiagramBlockCfg
      settings: OpenAtSimulationStart=off
  Real-Imag to Complex : RealImagToComplex
  Real-Imag to Complex1 : RealImagToComplex
  Unwrap : dspsigops/Unwrap  tol=pi  InputProcessing=Columns as channels (frame based)  running=on
  wires:
  Complex to Magnitude-Angle/2 -> Add/1
  Complex to Magnitude-Angle/1 -> Real-Imag to Complex/1, Real-Imag to Complex1/1
  Complex to Magnitude-Angle1/2 -> Add/2
  Unwrap/1 -> Real-Imag to Complex1/2
  Real-Imag to Complex1/1 -> HPA AM to PM/1
  In2/1 -> Complex to Magnitude-Angle1/1
  In1/1 -> Complex to Magnitude-Angle/1
  Add/1 -> Unwrap/1
  Complex to Magnitude-Angle1/1 -> Real-Imag to Complex/2
  Real-Imag to Complex/1 -> HPA AM to AM/1

== system Communication_Simulator/ISL Payload (SPARCS-B) /ISL/Input&Output of HPA1 ==
  In1 : Inport
  In2 : Inport  Port=2
  Add : Sum  Inputs=-+
  Complex to Magnitude-Angle : ComplexToMagnitudeAngle
  Complex to Magnitude-Angle1 : ComplexToMagnitudeAngle
  HPA AM to AM : ConstellationDiagram  Tag=ScatterPlot  WindowPosition=[1104 604 253 220]  SymbolsToDisplaySource=Property  SymbolsToDisplay=1000  Title=HPA AM to AM  XLimits=[-1.4713 6.1709]  YLimits=[-1.4713 6.1709]  XLabel=Input Amplitude  YLabel=Output Amplitude  ShowReferenceConstellation=off  ColorFading=on  DefaultConfigurationName=comm.scopes.ConstellationDiagramBlockCfg
      settings: OpenAtSimulationStart=off
  HPA AM to PM : ConstellationDiagram  Tag=ScatterPlot  WindowPosition=[842 605 253 220]  SymbolsToDisplaySource=Property  SymbolsToDisplay=1000  Title=HPA AM to PM  XLimits=[-1.0435 2.3201]  YLimits=[-1.0435 2.3201]  XLabel=Input Amplitude  YLabel=Phase Difference (rad)  ShowReferenceConstellation=off  ColorFading=on  DefaultConfigurationName=comm.scopes.ConstellationDiagramBlockCfg
      settings: OpenAtSimulationStart=off
  Real-Imag to Complex : RealImagToComplex
  Real-Imag to Complex1 : RealImagToComplex
  Unwrap : dspsigops/Unwrap  tol=pi  InputProcessing=Columns as channels (frame based)  running=on
  wires:
  Complex to Magnitude-Angle/2 -> Add/1
  Complex to Magnitude-Angle/1 -> Real-Imag to Complex/1, Real-Imag to Complex1/1
  Complex to Magnitude-Angle1/2 -> Add/2
  Unwrap/1 -> Real-Imag to Complex1/2
  Real-Imag to Complex1/1 -> HPA AM to PM/1
  In2/1 -> Complex to Magnitude-Angle1/1
  In1/1 -> Complex to Magnitude-Angle/1
  Add/1 -> Unwrap/1
  Complex to Magnitude-Angle1/1 -> Real-Imag to Complex/2
  Real-Imag to Complex/1 -> HPA AM to AM/1

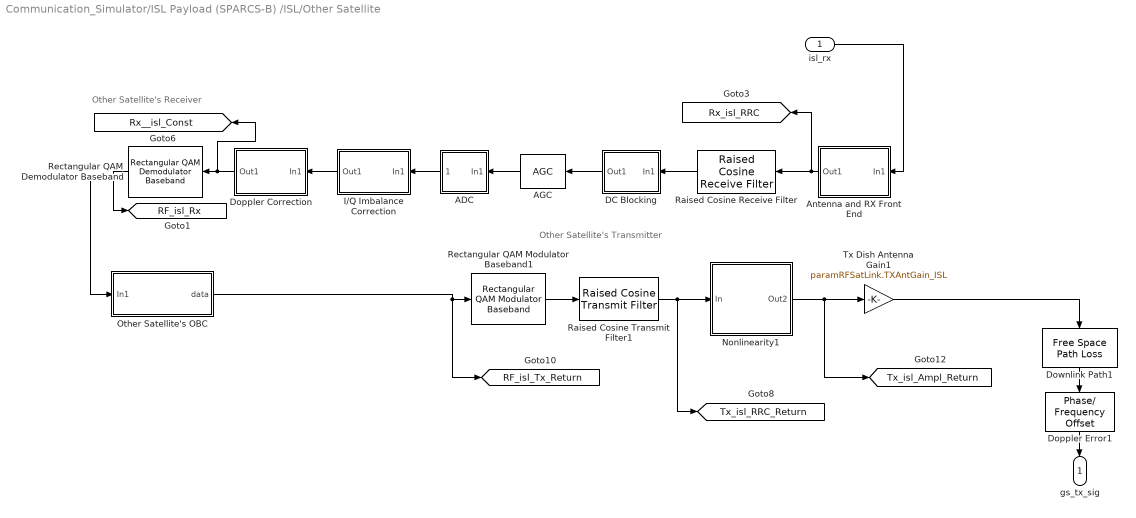
== system Communication_Simulator/ISL Payload (SPARCS-B) /ISL/Other Satellite ==
  note: Other Satellite's Transmitter
  note: Other Satellite's Receiver
  isl_rx : Inport
  ADC : Subsystem
      mask Display: disp('Bipolar\nADC')
  AGC : commrfcorlib/AGC  LegacyMode=off  DetectorMethod=Rectifier  LoopMethod=Linear  UpdatePeriod=100  StepSize=0.1  AdaptationStepSize=0.01  DesiredOutputPower=1  AveragingLength=256  MaximumGain=30  MaxPowerGain=400  GainOutputPort=off  InputPowerOutputPort=off  SimulateUsing=Code generation
  Antenna and RX Front End : Subsystem
      mask Display: disp('Antenna\nand\nRX Front End')
  DC Blocking : Subsystem
      mask Display: disp('DC\nBlocking')
  Doppler Correction : Subsystem
      mask Display: disp('Doppler\nCorrection')
  Doppler Error1 : commrflib2/Phase// Frequency Offset  phaseOffset=0  freqPort=off  freqOffset=paramRFSatLink.DoppOffset
  Downlink Path1 : commrflib2/Free Space Path Loss  mode=Distance and Frequency  dB=180  d=paramRFSatLink.Altitude  fc=paramRFSatLink.Frequency
  I/Q Imbalance Correction : Subsystem
      mask Display: disp('I/Q Imbalance\nCorrection')
  Nonlinearity1 : Subsystem
      mask Display: disp('HPA\n Nonlinearity\n with Optional\n Digital\nPredistortion')
  Other Satellite's OBC : Subsystem
  Raised Cosine Receive Filter : commfilt2/Raised Cosine Receive Filter  filtType=Square root  R=0.3  filtSpan=paramRFSatLink.FilterSpan  N=paramRFSatLink.SamplesPerSymbol  downFactor=paramRFSatLink.SamplesPerSymbol  downOffset=0  filterGain=1/sqrt(paramRFSatLink.SamplesPerSymbol)  InputProcessing=Columns as channels (frame based)  RateOptions=Enforce single-rate processing  framing=Mute  checkCoeff=off  variableName=rcRxFilt  currentFiltSpan=2*((2*(3))/2)  D=(2*(3))/2  inputOffset=0  sampMode=Mute  saveAsFlag=0  rateMode=Downsampling  checkGain=Normalized  launchFVT=off  roundingMode=Floor  overflowMode=off  coeffDataTypeStr=Inherit: Same word length as input  coeffMin=[]  coeffMax=[]  coeffLastDataTypeStr=Inherit: Same word length as input  accumDataTypeStr=Inherit: Same as product output  accumLastDataTypeStr=Inherit: Same as product output  outputDataTypeStr=Inherit: Same as accumulator  outputMin=[]  outputMax=[]  outputLastDataTypeStr=Inherit: Same as accumulator
  Raised Cosine Transmit Filter1 : commfilt2/Raised Cosine Transmit Filter  filtType=Square root  R=0.3  filtSpan=paramRFSatLink.FilterSpan  N=paramRFSatLink.SamplesPerSymbol  filterGain=sqrt(paramRFSatLink.SamplesPerSymbol)  InputProcessing=Columns as channels (frame based)  RateOptions=Enforce single-rate processing  framing=Mute  checkCoeff=off  variableName=rcTxFilt1  checkGain=Normalized  sampMode=Mute  saveAsFlag=0  currentFiltSpan=2*((2*(3))/2)  D=(2*(3))/2  launchFVT=off  roundingMode=Floor  overflowMode=off  coeffDataTypeStr=Inherit: Same word length as input  coeffMin=[]  coeffMax=[]  coeffLastDataTypeStr=Inherit: Same word length as input  outputDataTypeStr=Inherit: Same as accumulator  outputMin=[]  outputMax=[]  outputLastDataTypeStr=Inherit: Same as accumulator
  Rectangular QAM Demodulator Baseband : commdigbbndam3/Rectangular QAM Demodulator Baseband  M=16  OutType=Bit  DecType=Hard decision  VarSource=Dialog  Variance=1  Dec=Gray  Mapping=[0:15]  PowType=Average Power  MinDist=2  AvgPow=2  PeakPow=1  Ph=0  outDtype1=double  outDtype2=double  derotateFactorWordLen=16  derotateFactorDataTypeStr=Inherit: Same word length as input  derotateFactorLastDataTypeStr=Inherit: Same word length as input  denormFactorWordLen=16  denormFactorDataTypeStr=Inherit: Same word length as input  denormFactorLastDataTypeStr=Inherit: Same word length as input  prodOutWordLen=32  prodOutOverflowMode=Wrap  prodOutRoundingMode=Floor  prodOutOvFlMode=off  prodOutOvFlModeLastStrValue=off  sumWordLen=32
  Rectangular QAM Modulator Baseband1 : commdigbbndam3/Rectangular QAM Modulator Baseband  M=16  InType=Bit  Enc=Gray  Mapping=[0:15]  PowType=Average Power  MinDist=2  AvgPow=1  PeakPow=1  Ph=0  outDtype=double  outWordLen=16  outUDDataType=sfix(16)  outFracLenMode=Best precision  outFracLen=15  outDataTypeStr=double  outLastDataTypeStr=double
  Tx Dish Antenna Gain1 : Gain  Gain=paramRFSatLink.TXAntGain_ISL  SaturateOnIntegerOverflow=on  OutDataTypeStr=Inherit: Same as input  ParamDataTypeStr=Inherit: Same as input
  gs_tx_sig : Outport
  tag scope: RF_isl_Rx=global, RF_isl_Tx_Return=global, Rx__isl_Const=global, Rx_isl_RRC=global, Tx_isl_Ampl_Return=global, Tx_isl_RRC_Return=global
  wires:
  Doppler Error1/1 -> gs_tx_sig/1
  Downlink Path1/1 -> Doppler Error1/1
  Tx Dish Antenna Gain1/1 -> Downlink Path1/1
  Rectangular QAM Modulator Baseband1/1 -> Raised Cosine Transmit Filter1/1
  Nonlinearity1/1(Out2) -> Tx Dish Antenna Gain1/1, [Tx_isl_Ampl_Return]
  Raised Cosine Transmit Filter1/1 -> Nonlinearity1/1(In), [Tx_isl_RRC_Return]
  Other Satellite's OBC/1(data) -> [RF_isl_Tx_Return], Rectangular QAM Modulator Baseband1/1
  I/Q Imbalance Correction/1(Out1) -> Doppler Correction/1(In1)
  Antenna and RX Front End/1(Out1) -> [Rx_isl_RRC], Raised Cosine Receive Filter/1
  DC Blocking/1(Out1) -> AGC/1
  ADC/1(Out2) -> I/Q Imbalance Correction/1(In1)
  Doppler Correction/1(Out1) -> Rectangular QAM Demodulator Baseband/1, [Rx__isl_Const]
  AGC/1 -> ADC/1(In1)
  isl_rx/1 -> Antenna and RX Front End/1(In1)
  Raised Cosine Receive Filter/1 -> DC Blocking/1(In1)
  Rectangular QAM Demodulator Baseband/1 -> [RF_isl_Rx], Other Satellite's OBC/1(In1)

== system Communication_Simulator/ISL Payload (SPARCS-B) /ISL/Power Spectrum ==
  In1 : Inport
  In2 : Inport  Port=2
  Matrix Concatenation : Concatenate  Mode=Multidimensional array  ConcatenateDimension=2
  Tx and Rx Spectrum : SpectrumAnalyzer  WindowPosition=[258.000000,231.000000,1020.000000,403.000000,]  ScopeFrameLocation=window  Method=Welch  SampleRate=200000  Span=200000  StartFrequency=-100000  StopFrequency=100000  AveragingMethod=Running  YLimits=[-153.17824983,37.77721687]  ShowLegend=on  ChannelNames="[\"Tramsitted \",\"Received\"]"  SelectedToolstripTab=spectrumAnalyzerToolstrip.spectrumTab  AllowFFTLengthLessThanSamplesPerUpdate=on  DefaultConfigurationName=spbscopes.SpectrumAnalyzerBlockCfg  IsFrequencyInputMode=0  FrequencyVectorPort=0  FrequencyVectorFromPort=0  FrequencyInputRBWPort=0  FrequencyInputRBWFromPort=0
  wires:
  Matrix Concatenation/1 -> Tx and Rx Spectrum/1
  In2/1 -> Matrix Concatenation/2
  In1/1 -> Matrix Concatenation/1

== system Communication_Simulator/ISL Payload (SPARCS-B) /ISL/Power Spectrum1 ==
  In1 : Inport
  In2 : Inport  Port=2
  Matrix Concatenation : Concatenate  Mode=Multidimensional array  ConcatenateDimension=2
  Tx and Rx Spectrum : SpectrumAnalyzer  WindowPosition=[25 331 480 288]  Method=Welch  SampleRate=200000  Span=200000  StartFrequency=-100000  StopFrequency=100000  AveragingMethod=Running  YLimits=[-90.208205220815884218,27.456041881558888917]  ShowLegend=on  ChannelNames="[\"Tramsitted \",\"Received\"]"  AllowFFTLengthLessThanSamplesPerUpdate=on  DefaultConfigurationName=spbscopes.SpectrumAnalyzerBlockCfg  IsFrequencyInputMode=0  FrequencyVectorPort=0  FrequencyVectorFromPort=0  FrequencyInputRBWPort=0  FrequencyInputRBWFromPort=0
      settings: OpenAtSimulationStart=off
  wires:
  Matrix Concatenation/1 -> Tx and Rx Spectrum/1
  In2/1 -> Matrix Concatenation/2
  In1/1 -> Matrix Concatenation/1

== system Communication_Simulator/ISL Payload (SPARCS-B) /ISL/Subsystem ==

== system Communication_Simulator/ISL Payload (SPARCS-B) /ISL/Subsystem1 ==

== system Communication_Simulator/ISL Payload (SPARCS-B) /ISL/background11 ==

== system Communication_Simulator/ISL Payload (SPARCS-B) /ISL/background12 ==

== system Communication_Simulator/ISL Payload (SPARCS-B) /ISL/background13 ==

== system Communication_Simulator/ISL Payload (SPARCS-B) /ISL/background14 ==

== system Communication_Simulator/ISL Payload (SPARCS-B) /ISL/background4 ==

== system Communication_Simulator/ISL Payload (SPARCS-B) /ISL/background5 ==

== system Communication_Simulator/ISL Payload (SPARCS-B) /ISL/background6 ==

== system Communication_Simulator/ISL Payload (SPARCS-B) /ISL/background7 ==
